simulink subsystem "TimeSubscriber"  (R2022b)
settings: Solver=VariableStepAuto  StartTime=0.0  StopTime=10.0  RelTol=1e-3
libraries: ros2lib x1
settings Model: Creator=hollis  LastModifiedBy=hollis

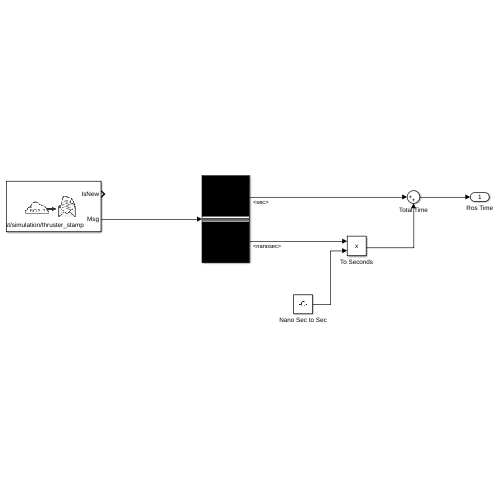
[thumbnail: Simulink's stored preview of the top-level diagram]
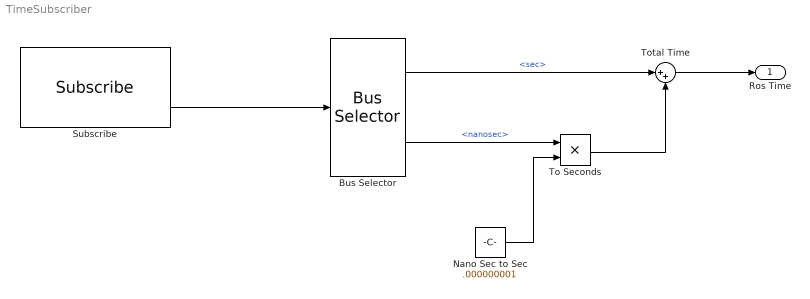
== system TimeSubscriber ==
  Bus Selector : BusSelector  OutputSignals=stamp.sec,stamp.nanosec
  Nano Sec to Sec : Constant  Value=.000000001
  Subscribe : ros2lib/Subscribe  topicSource=Select from ROS network  topic=/tempest/simulation/thruster_stamp  messageType=std_msgs/Header  sampleTime=-1  QOSHistory=Keep last  QOSDepth=1  QOSReliability=Reliable  QOSDurability=Volatile
      settings: LibrarySourceBlock=roslib/ROS 2/Subscribe
  To Seconds : Product
  Total Time : Sum  Inputs=|++
  Ros Time : Outport
  wires:
  Subscribe/2 -> Bus Selector/1
  Bus Selector/2 -> To Seconds/1  "<nanosec>"
  Nano Sec to Sec/1 -> To Seconds/2
  Bus Selector/1 -> Total Time/1  "<sec>"
  To Seconds/1 -> Total Time/2
  Total Time/1 -> Ros Time/1
